simulink model "LAB_02_26_SEPT_SIM_2BODYDYN"  (R2022b)
settings: Solver=VariableStepAuto  StartTime=t0  StopTime=tf  RelTol=1e-3
values from neighbouring files (symbols this model uses):
  mu_sun = 1.327e+11    (= 132700000000)    [LAB_02_26_SEPT_MAT_2BODYDYN.m]
  r0 = [2.029e+8; -1.475e+5; -1.1395e+7]    [LAB_02_26_SEPT_MAT_2BODYDYN.m]
  v0 = [3.021; 24.139; 10.964]    [LAB_02_26_SEPT_MAT_2BODYDYN.m]    (also in LAB_02_26_SEPT_MAT_SMD.m = 0)
settings Model: Creator=maria  LastModifiedBy=maria

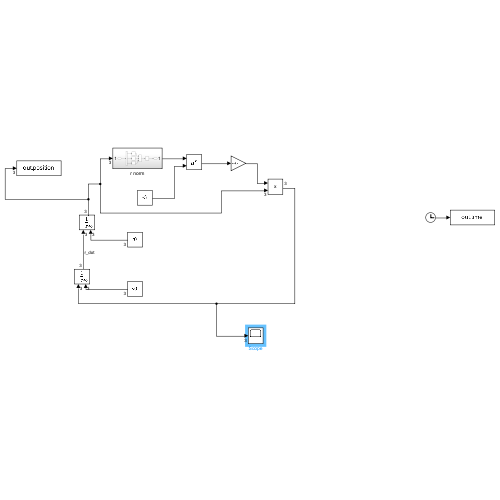
[thumbnail: Simulink's stored preview of the top-level diagram]
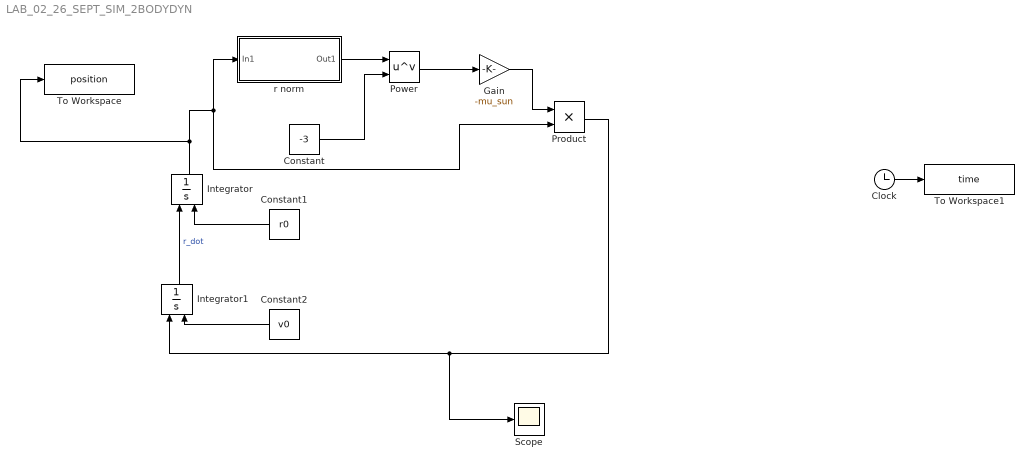
== system LAB_02_26_SEPT_SIM_2BODYDYN ==
  Clock : Clock
  Constant : Constant  Value=-3
  Constant1 : Constant  Value=r0
  Constant2 : Constant  Value=v0
  Gain : Gain  Gain=-mu_sun
  Integrator : Integrator  InitialConditionSource=external
  Integrator1 : Integrator  InitialConditionSource=external
  Power : Math  Operator=pow
  Product : Product
  Scope : Scope
  To Workspace : ToWorkspace  VariableName=position  SaveFormat=Timeseries  SampleTime=-1
  To Workspace1 : ToWorkspace  VariableName=time  SaveFormat=Timeseries  SampleTime=-1
  r norm : Subsystem
  wires:
  r norm/1(Out1) -> Power/1
  Constant/1 -> Power/2
  Power/1 -> Gain/1
  Integrator/1 -> To Workspace/1, r norm/1(In1), Product/2
  Integrator1/1 -> Integrator/1  "r_dot"
  Constant1/1 -> Integrator/2
  Constant2/1 -> Integrator1/2
  Gain/1 -> Product/1
  Product/1 -> Scope/1, Integrator1/1
  Clock/1 -> To Workspace1/1

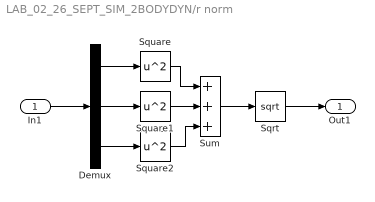
== system LAB_02_26_SEPT_SIM_2BODYDYN/r norm ==
  In1 : Inport
  Demux : Demux  Outputs=3
  Sqrt : Sqrt
  Square : Math  Operator=square
  Square1 : Math  Operator=square
  Square2 : Math  Operator=square
  Sum : Sum  Inputs=+++
  Out1 : Outport
  wires:
  Demux/1 -> Square/1
  Demux/2 -> Square1/1
  Demux/3 -> Square2/1
  Sum/1 -> Sqrt/1
  Sqrt/1 -> Out1/1
  Square/1 -> Sum/1
  Square1/1 -> Sum/2
  Square2/1 -> Sum/3
  In1/1 -> Demux/1
